simulink model "problem1_block"  (R2024b)
settings: Solver=ode4  StartTime=0.0  StopTime=10  FixedStep=0.00018919  RelTol=1e-3
values from neighbouring files (symbols this model uses):
  P_s = 13.8e6    (= 13800000)    [problem1.m]
  Q_max = 2.5e-4    (= 0.00025)    [problem1.m]
undefined symbols (not defined in the file or in its folder): den_dG1, den_dG2, den_dv, den_dx, num_dG1, num_dG2, num_dv, num_dx
settings Model: Creator=piero  LastModifiedBy=piero

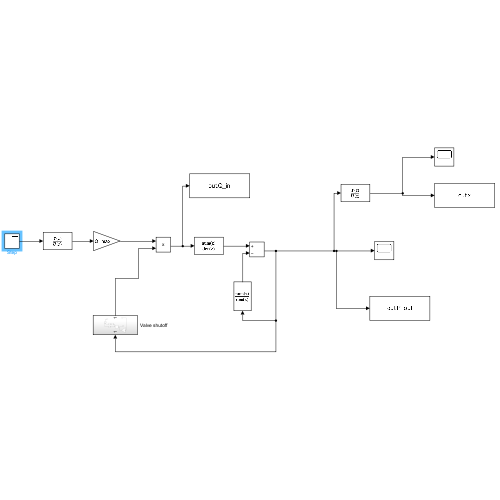
[thumbnail: Simulink's stored preview of the top-level diagram]
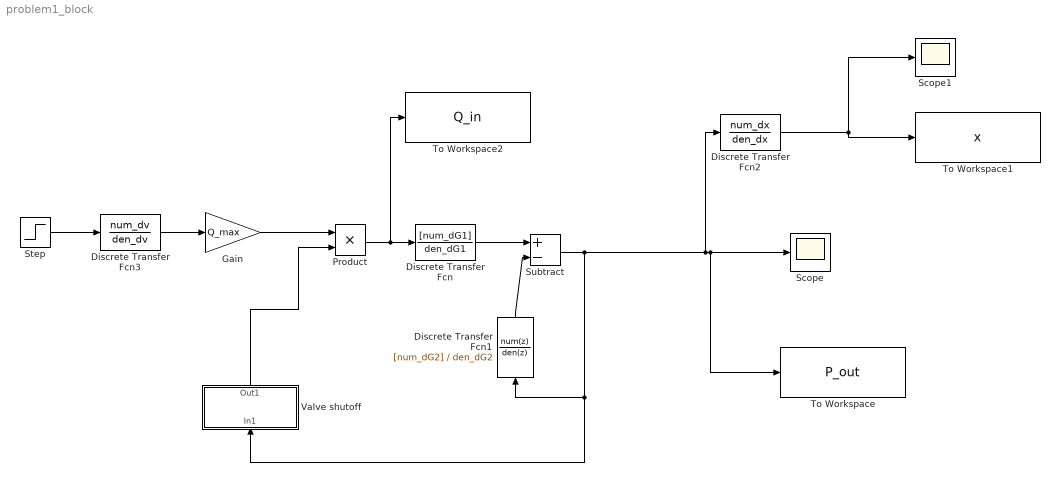
== system problem1_block ==
  Discrete Transfer Fcn : DiscreteTransferFcn  Numerator=[num_dG1]  Denominator=den_dG1
  Discrete Transfer Fcn1 : DiscreteTransferFcn  Numerator=[num_dG2]  Denominator=den_dG2
  Discrete Transfer Fcn2 : DiscreteTransferFcn  Numerator=num_dx  Denominator=den_dx
  Discrete Transfer Fcn3 : DiscreteTransferFcn  Numerator=num_dv  Denominator=den_dv
  Gain : Gain  Gain=Q_max
  Product : Product
  Scope : Scope
  Scope1 : Scope
  Step : Step  Time=0.1  SampleTime=0
  Subtract : Sum  Inputs=+-
  To Workspace : ToWorkspace  VariableName=P_out  SaveFormat=Timeseries  SampleTime=-1
  To Workspace1 : ToWorkspace  VariableName=x  SaveFormat=Timeseries  SampleTime=-1
  To Workspace2 : ToWorkspace  VariableName=Q_in  SaveFormat=Timeseries  SampleTime=-1
  "Valve shutoff " : Subsystem
  wires:
  Step/1 -> Discrete Transfer Fcn3/1
  Gain/1 -> Product/1
  Product/1 -> Discrete Transfer Fcn/1, To Workspace2/1
  Discrete Transfer Fcn/1 -> Subtract/1
  Discrete Transfer Fcn1/1 -> Subtract/2
  "Valve shutoff "/1(Out1) -> Product/2
  Subtract/1 -> Discrete Transfer Fcn2/1, To Workspace/1, Scope/1, Discrete Transfer Fcn1/1, "Valve shutoff "/1(In1)
  Discrete Transfer Fcn2/1 -> To Workspace1/1, Scope1/1
  Discrete Transfer Fcn3/1 -> Gain/1

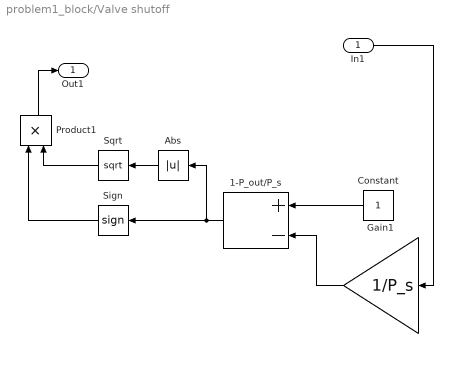
== system problem1_block/Valve shutoff  ==
  In1 : Inport
  1-P_out/P_s : Sum  Inputs=+-
  Abs : Abs  SaturateOnIntegerOverflow=off
  Constant : Constant
  Gain1 : Gain  Gain=1/P_s
  Product1 : Product
  Sign : Signum
  Sqrt : Sqrt
  Out1 : Outport
  wires:
  Constant/1 -> 1-P_out/P_s/1
  1-P_out/P_s/1 -> Sign/1, Abs/1
  Gain1/1 -> 1-P_out/P_s/2
  Sqrt/1 -> Product1/2
  Abs/1 -> Sqrt/1
  Sign/1 -> Product1/1
  In1/1 -> Gain1/1
  Product1/1 -> Out1/1
